simulink model "sesion2_act1"  (R2021a)
settings: Solver=ode1  StartTime=0.0  StopTime=10.0  FixedStep=0.001  RelTol=1e-3
values from neighbouring files (symbols this model uses):
  a = 1    [sesion2.m]
  b = 1    [sesion2.m]
settings Model: Creator=valen  LastModifiedBy=valen
settings DataIOCC: SaveFormat=Structure

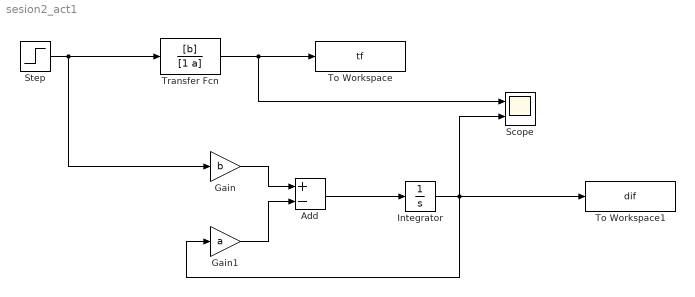
== system sesion2_act1 ==
  Add : Sum  Inputs=+-
  Gain : Gain  Gain=b
  Gain1 : Gain  Gain=a
  Integrator : Integrator
  Scope : Scope  NumInputPorts=2
  Step : Step  SampleTime=0
  To Workspace : ToWorkspace  VariableName=tf  SampleTime=-1
  To Workspace1 : ToWorkspace  VariableName=dif  SampleTime=-1
  Transfer Fcn : TransferFcn  Numerator=[b]  Denominator=[1 a]
  wires:
  Step/1 -> Gain/1, Transfer Fcn/1
  Transfer Fcn/1 -> Scope/1, To Workspace/1
  Gain/1 -> Add/1
  Gain1/1 -> Add/2
  Add/1 -> Integrator/1
  Integrator/1 -> Gain1/1, To Workspace1/1, Scope/2
